simulink model "Power_Model_Official_Pars_2022a"  (R2022a)
settings: Solver=ode23t  StartTime=0.0  StopTime=500  RelTol=1e-3
values from neighbouring files (symbols this model uses):
  anode_tube_D = 0.01    [fuel_cell_battery_par.mat]
  cathode_tube_D = 0.05    [fuel_cell_battery_par.mat]
  comp_rpm_TLU = [0 1800 3600]    [fuel_cell_battery_par.mat]
  coolant_num_layers = 20    [fuel_cell_battery_par.mat]
  coolant_num_passes = 12    [fuel_cell_battery_par.mat]
  coolant_tube_D = 0.05    [fuel_cell_battery_par.mat]
  coolant_w_channels = 1    [fuel_cell_battery_par.mat]
  env_p = 0.101325    [fuel_cell_battery_par.mat]
  env_T = 20    [fuel_cell_battery_par.mat]
  env_yH20 = 0.0115436377169    [fuel_cell_battery_par.mat]
  env_yO2 = 0.21    [fuel_cell_battery_par.mat]
  radiator_air_area_fins = 11.5625    [fuel_cell_battery_par.mat]
  radiator_air_area_primary = 1.223125    [fuel_cell_battery_par.mat]
  radiator_eta_fin = 0.7    [fuel_cell_battery_par.mat]
  radiator_N_tubes = 25    [fuel_cell_battery_par.mat]
  radiator_rho = 2700    [fuel_cell_battery_par.mat]
  radiator_t_wall = 0.0001    [fuel_cell_battery_par.mat]
  radiator_tube_H = 0.0015    [fuel_cell_battery_par.mat]
  radiator_W = 0.025    [fuel_cell_battery_par.mat]
  stack_area = 280    [fuel_cell_battery_par.mat]
  stack_iL = 1.4    [fuel_cell_battery_par.mat]
  stack_mea_rho = 1800    [fuel_cell_battery_par.mat]
  stack_num_cells = 400    [fuel_cell_battery_par.mat]
  stack_num_channels = 8    [fuel_cell_battery_par.mat]
  stack_t_gdl = 250    [fuel_cell_battery_par.mat]
  stack_t_membrane = 125    [fuel_cell_battery_par.mat]
  stack_w_channels = 1    [fuel_cell_battery_par.mat]
undefined symbols (not defined in the file or in its folder): Bat, BattCapInit, BattChargeMax, BattTempBp, CapLUTBp, CapSOCBp, Em, f_fc_auxpower, f_fc_currcmd_bpt, f_fc_h2flow, f_fc_heatflow, f_fc_tmpcmd_bpt, f_fc_voltage, Mot, Np, Ns, RInt, Tc_Batt
libraries: fl_lib x89, nesl_utility x39, FuelCell_lib x32, ee_lib x3, slpidlib x3, batteryecm_lib x1, simulink_extras x1, autolibshared x1, simulink x1
(part 4 of 4)

== system Power_Model_Official_Pars_2022a/Fuel Cell/Fuel Cell/Simscape Fuel Cell_2/Hydrogen Source ==
  Constant1 : Constant  Value=env_p
  Fuel Tank : FuelCell_lib/elements/Constant Volume Chamber (FC)  V0=tank_V l  num_ports=foundation.enum.num_ports.one  area_A=0.01 m^2  area_B=0.01 m^2  area_C=0.01 m^2  area_D=0.01 m^2  cond_spec=FuelCell.enum.ChamberCondSpec.Enabled  tau_c=1 s  is_cond=[0; 0; 0; 0]  out_comp=FuelCell.enum.Composition.Mole  p0=tank_p MPa  T0=env_T degC  comp=FuelCell.enum.Composition.Mole  y0=[0; 0; 1; 0]  x0=[1; 0; 0; 0]
      settings: InternalSimscapePortConfiguration="{\"Bottom\":[{\"id\":\"H\",\"label\":\"H\",\"type\":\"foundation.thermal.thermal\"}],\"Left\":[{\"id\":\"MIn\",\"label\":\"MIn\",\"type\":\"input\"},{\"id\":\"TIn\",\"label\":\"TIn\",\"type\":\"input\"}],\"Right\":[{\"id\":\"pC\",\"label\":\"p\",\"type\":\"output\"},{\"id\":\"TC\",\"label\":\"T\",\"type\":\"output\"},{\"id\":\"yC_i\",\"label\":\"y_i\",\"type\":\"output\"}],\"Top\":[{\"id\":\"A\",\"label\":\"A\",\"type\":\"FuelCell.FuelCell\"}]}"
  Perfect Insulator : fl_lib/Thermal/Thermal Elements/Perfect Insulator  T_specify=off  T_priority=None  T=0 K  T_nominal_specify=off  T_nominal_unit=K  T_nominal_value=1
  Perfect Insulator1 : fl_lib/Thermal/Thermal Elements/Perfect Insulator  T_specify=off  T_priority=None  T=0 K  T_nominal_specify=off  T_nominal_unit=K  T_nominal_value=1
  Pipe (FC) : FuelCell_lib/elements/Pipe (FC)  length=1 m  area=pi*anode_tube_D^2/4 m^2  Dh=anode_tube_D m  extra_length=0.1 * 100 m  roughness=15e-6 m  Re_lam=2000  Re_tur=4000  shape_factor=64  Nu_lam=3.66  tau_c=1e-3 s  isCond=[0; 0; 0; 0]  volMeas=false  compMeas=FuelCell.enum.Composition.Mole  p0=env_p MPa  T0=env_T degC  comp=FuelCell.enum.Composition.Mole  y0=[0; 0; 1; 0]  x0=[1; 0; 0; 0]
      settings: InternalSimscapePortConfiguration="{\"Bottom\":[{\"id\":\"MIn\",\"label\":\"M_in\",\"type\":\"input\"},{\"id\":\"TIn\",\"label\":\"T_in\",\"type\":\"input\"}],\"Left\":[{\"id\":\"A\",\"label\":\"A\",\"type\":\"FuelCell.FuelCell\"},{\"id\":\"H\",\"label\":\"H\",\"type\":\"foundation.thermal.thermal\"}],\"Right\":[{\"id\":\"B\",\"label\":\"B\",\"type\":\"FuelCell.FuelCell\"}],\"Top\":[]}"
  Pressure-Reducing Valve : Subsystem  Tag=PublishSubsystem  mask(Pressure-Reducing Valve){D=anode_tube_D, r_min=1e-4, r_max=0.2, p_range=0.005}
      mask prompts: D "Connecting tube diameter (m)"; r_min "Min diameter ratio"; r_max "Max diameter ratio"; p_range "Pressure regulation range (MPa)"
      mask help: This subsystem models a pressure reducing valve that maintains a set pressure at port B. The valve is normally open. When the pressure is above the set pressure, it is fully closed.
  Simulink-PS Converter : nesl_utility/Simulink-PS Converter  PhysicalDomain=network_engine_domain  SubClassName=ps_input  LeftPortType=input  RightPortType=output  PseudoPeriodic=off  Frequencies=[]  NoiseDistribution=none  NoiseParameters=[]  Unit=MPa  AffineConversion=off  FilteringAndDerivatives=provide  SimscapeFilterOrder=1  InputFilterTimeConstant=0.001  UdotUserProvided=0
  Stack Pressure : Constant  Value=0.06
  Sum : Sum  Inputs=++|
  H2 : PMIOPort  Side=Right
  wires:
  Sum/1 -> Simulink-PS Converter/1
  Constant1/1 -> Sum/2
  Stack Pressure/1 -> Sum/1
  connections:
  Perfect Insulator/LConn1 -- Fuel Tank/RConn4
  Fuel Tank/LConn3 -- Pressure-Reducing Valve/LConn1
  Pressure-Reducing Valve/RConn1 -- Pipe (FC)/LConn1
  Pipe (FC)/RConn1 -- H2/RConn1
  Perfect Insulator1/LConn1 -- Pipe (FC)/LConn2
  Simulink-PS Converter/RConn1 -- Pressure-Reducing Valve/LConn2

== system Power_Model_Official_Pars_2022a/Fuel Cell/Fuel Cell/Simscape Fuel Cell_2/Measurements ==
  Gain : Gain  Gain=1e-3
  Mux : Mux  Inputs=2
  Product : Product
  i : Outport
  v : Outport  Port=2
  P : Outport  Port=3
  T : Outport  Port=4
  wires:
  [v_stack] -> Product/2, v/1
  [i_stack] -> Product/1, i/1
  [T_stack] -> T/1
  [Q_stack] -> Mux/2
  Product/1 -> Gain/1
  Mux/1 -> P/1
  Gain/1 -> Mux/1

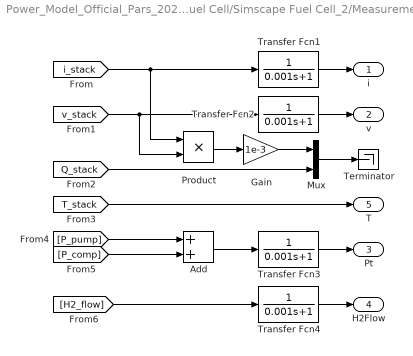
== system Power_Model_Official_Pars_2022a/Fuel Cell/Fuel Cell/Simscape Fuel Cell_2/Measurements1 ==
  Add : Sum
  Gain : Gain  Gain=1e-3
  Mux : Mux  Inputs=2
  Product : Product
  Terminator : Terminator
  Transfer Fcn{1..4} (4 alike) : TransferFcn  Denominator=[0.001 1]
  i : Outport
  v : Outport  Port=2
  Pt : Outport  Port=3
  H2Flow : Outport  Port=4
  T : Outport  Port=5
  wires:
  Gain/1 -> Mux/1
  Mux/1 -> Terminator/1
  Product/1 -> Gain/1
  [Q_stack] -> Mux/2
  [T_stack] -> T/1
  [i_stack] -> Transfer Fcn1/1, Product/1
  [v_stack] -> Transfer Fcn2/1, Product/2
  Transfer Fcn1/1 -> i/1
  Transfer Fcn2/1 -> v/1
  [P_pump] -> Add/1
  [P_comp] -> Add/2
  Add/1 -> Transfer Fcn3/1
  Transfer Fcn3/1 -> Pt/1
  [H2_flow] -> Transfer Fcn4/1
  Transfer Fcn4/1 -> H2Flow/1

== system Power_Model_Official_Pars_2022a/Fuel Cell/Fuel Cell/Simscape Fuel Cell_2/Oxygen Source ==
  i_cmd : Inport
  Air Intake : FuelCell_lib/elements/Reservoir (FC)  constCond=true  p0=env_p MPa  T0=env_T degC  comp=FuelCell.enum.Composition.Mole  y0=[1-env_yO2-env_yH20; env_yO2; 0; env_yH20]  x0=[1; 0; 0; 0]  area=pi*cathode_tube_D^2/4 m^2
      settings: InternalSimscapePortConfiguration="{\"Bottom\":[],\"Left\":[],\"Right\":[],\"Top\":[{\"id\":\"A\",\"label\":\"A\",\"type\":\"FuelCell.FuelCell\"}]}"
  Compressor : FuelCell_lib/sources/Mass Flow Rate Source (FC)  source_type=foundation.enum.constant_controlled.controlled  flow_rate=0 kg/s  power_spec=foundation.enum.power_spec.isentropic  area_A=pi*cathode_tube_D^2/4 m^2  area_B=pi*cathode_tube_D^2/4 m^2  mdot_A_specify=off  mdot_A_priority=None  mdot_A=0.1 kg/s  mdot_A_nominal_specify=off  mdot_A_nominal_unit=kg/s  mdot_A_nominal_value=1  mdot_B_specify=off  mdot_B_priority=None  mdot_B=0.1 kg/s  mdot_B_nominal_specify=off  mdot_B_nominal_unit=kg/s  mdot_B_nominal_value=1  phi_A_specify=off  phi_A_priority=None  phi_A=0 J/s  phi_A_nominal_specify=off  phi_A_nominal_unit=J/s  phi_A_nominal_value=1  phi_B_specify=off  phi_B_priority=None  phi_B=0 J/s  phi_B_nominal_specify=off  phi_B_nominal_unit=J/s  phi_B_nominal_value=1  mdot_A_i_specify=off  mdot_A_i_priority=None  mdot_A_i=[0; 0; 0; 0] kg/s  mdot_A_i_nominal_specify=off  mdot_A_i_nominal_unit=kg/s  mdot_A_i_nominal_value=1  mdot_B_i_specify=off  mdot_B_i_priority=None  mdot_B_i=[0; 0; 0; 0] kg/s  mdot_B_i_nominal_specify=off  mdot_B_i_nominal_unit=kg/s  mdot_B_i_nominal_value=1
      settings: InternalSimscapePortConfiguration="{\"Bottom\":[],\"Left\":[{\"id\":\"M\",\"label\":\"M\",\"type\":\"input\"},{\"id\":\"A\",\"label\":\"A\",\"type\":\"FuelCell.FuelCell\"}],\"Right\":[{\"id\":\"B\",\"label\":\"B\",\"type\":\"FuelCell.FuelCell\"}],\"Top\":[]}"
  Compressor Volume : FuelCell_lib/elements/Constant Volume Chamber (FC)  V0=0.3 l  num_ports=foundation.enum.num_ports.two  area_A=pi*cathode_tube_D^2/4 m^2  area_B=pi*cathode_tube_D^2/4 m^2  area_C=0.01 m^2  area_D=0.01 m^2  cond_spec=FuelCell.enum.ChamberCondSpec.Enabled  tau_c=1e-3 s  is_cond=[0; 0; 0; 0]  out_comp=FuelCell.enum.Composition.Mole  p0=env_p MPa  T0=env_T degC  comp=FuelCell.enum.Composition.Mole  y0=[1-env_yO2-env_yH20; env_yO2; 0; env_yH20]  x0=[1; 0; 0; 0]
      settings: InternalSimscapePortConfiguration="{\"Bottom\":[{\"id\":\"H\",\"label\":\"H\",\"type\":\"foundation.thermal.thermal\"}],\"Left\":[{\"id\":\"MIn\",\"label\":\"MIn\",\"type\":\"input\"},{\"id\":\"TIn\",\"label\":\"TIn\",\"type\":\"input\"}],\"Right\":[{\"id\":\"pC\",\"label\":\"p\",\"type\":\"output\"},{\"id\":\"TC\",\"label\":\"T\",\"type\":\"output\"},{\"id\":\"yC_i\",\"label\":\"y_i\",\"type\":\"output\"}],\"Top\":[{\"id\":\"A\",\"label\":\"A\",\"type\":\"FuelCell.FuelCell\"},{\"id\":\"B\",\"label\":\"B\",\"type\":\"FuelCell.FuelCell\"}]}"
  Compressor Control : Subsystem
  Compressor Map : Subsystem
  Mass Flow Rate Sensor (FC) : FuelCell_lib/sensors/Mass Flow Rate Sensor (FC)
      settings: InternalSimscapePortConfiguration="{\"Bottom\":[],\"Left\":[{\"id\":\"A\",\"label\":\"A\",\"type\":\"FuelCell.FuelCell\"}],\"Right\":[{\"id\":\"M\",\"label\":\"M\",\"type\":\"output\"},{\"id\":\"Phi_out\",\"label\":\"Phi\",\"type\":\"output\"},{\"id\":\"M_i\",\"label\":\"M_i\",\"type\":\"output\"},{\"id\":\"B\",\"label\":\"B\",\"type\":\"FuelCell.FuelCell\"}],\"Top\":[]}"
  Max rpm : fl_lib/Physical Signals/Functions/PS Gain  gain=max(comp_rpm_TLU) rpm
  Oxygen Excess Ratio : Constant  Value=2.5
  PS-Simulink Converter : nesl_utility/PS-Simulink Converter  PhysicalDomain=network_engine_domain  SubClassName=ps_output  LeftPortType=input  RightPortType=output  PseudoPeriodic=off  Frequencies=[]  VectorFormat=1-D array  Unit=kg/s  AffineConversion=off
  Perfect Insulator : fl_lib/Thermal/Thermal Elements/Perfect Insulator  T_specify=off  T_priority=None  T=0 K  T_nominal_specify=off  T_nominal_unit=K  T_nominal_value=1
  Simulink-PS Converter : nesl_utility/Simulink-PS Converter  PhysicalDomain=network_engine_domain  SubClassName=ps_input  LeftPortType=input  RightPortType=output  PseudoPeriodic=off  Frequencies=[]  NoiseDistribution=none  NoiseParameters=[]  Unit=1  AffineConversion=off  FilteringAndDerivatives=provide  SimscapeFilterOrder=1  InputFilterTimeConstant=0.001  UdotUserProvided=0
  O2 : PMIOPort  Side=Left
  wires:
  Compressor Control/1(cmd) -> Simulink-PS Converter/1
  i_cmd/1 -> Compressor Control/2(i)
  PS-Simulink Converter/1 -> Compressor Control/3(M_meas)
  Oxygen Excess Ratio/1 -> Compressor Control/1(OER)
  connections:
  Compressor Map/RConn3 -- Compressor/RConn1 -- Compressor Volume/LConn4
  Compressor Map/RConn1 -- Compressor/LConn2 -- Air Intake/LConn1
  Compressor/LConn1 -- Compressor Map/LConn1
  Simulink-PS Converter/RConn1 -- Max rpm/LConn1
  Max rpm/RConn1 -- Compressor Map/RConn2
  O2/RConn1 -- Mass Flow Rate Sensor (FC)/RConn4
  PS-Simulink Converter/LConn1 -- Mass Flow Rate Sensor (FC)/RConn1
  Compressor Volume/RConn4 -- Perfect Insulator/LConn1
  Compressor Volume/LConn3 -- Mass Flow Rate Sensor (FC)/LConn1

== system Power_Model_Official_Pars_2022a/Fuel Cell/Fuel Cell/Simscape Fuel Cell_2/Recirculation ==
  Constant Volume Chamber (FC) : FuelCell_lib/elements/Constant Volume Chamber (FC)  V0=0.05^3 m^3  num_ports=foundation.enum.num_ports.three  area_A=pi*anode_tube_D^2/4 m^2  area_B=pi*anode_tube_D^2/4 m^2  area_C=pi*anode_tube_D^2/4 m^2  area_D=0.01 m^2  cond_spec=FuelCell.enum.ChamberCondSpec.Enabled  tau_c=1e-3 s  is_cond=[0; 0; 0; 0]  out_comp=FuelCell.enum.Composition.Mole  p0=env_p MPa  T0=env_T degC  comp=FuelCell.enum.Composition.Mole  y0=[0; 0; 1; 0]  x0=[1; 0; 0; 0]
      settings: InternalSimscapePortConfiguration="{\"Bottom\":[{\"id\":\"H\",\"label\":\"H\",\"type\":\"foundation.thermal.thermal\"}],\"Left\":[{\"id\":\"MIn\",\"label\":\"MIn\",\"type\":\"input\"},{\"id\":\"TIn\",\"label\":\"TIn\",\"type\":\"input\"}],\"Right\":[{\"id\":\"pC\",\"label\":\"p\",\"type\":\"output\"},{\"id\":\"TC\",\"label\":\"T\",\"type\":\"output\"},{\"id\":\"yC_i\",\"label\":\"y_i\",\"type\":\"output\"}],\"Top\":[{\"id\":\"A\",\"label\":\"A\",\"type\":\"FuelCell.FuelCell\"},{\"id\":\"B\",\"label\":\"B\",\"type\":\"FuelCell.FuelCell\"},{\"id\":\"C\",\"label\":\"C\",\"type\":\"FuelCell.FuelCell\"}]}"
  Feedforward Control : Subsystem
  Mass Flow Rate Source (FC) : FuelCell_lib/sources/Mass Flow Rate Source (FC)  source_type=foundation.enum.constant_controlled.controlled  flow_rate=0 kg/s  power_spec=foundation.enum.power_spec.none  area_A=0.01 m^2  area_B=0.01 m^2  mdot_A_specify=off  mdot_A_priority=None  mdot_A=0.1 kg/s  mdot_A_nominal_specify=off  mdot_A_nominal_unit=kg/s  mdot_A_nominal_value=1  mdot_B_specify=off  mdot_B_priority=None  mdot_B=0.1 kg/s  mdot_B_nominal_specify=off  mdot_B_nominal_unit=kg/s  mdot_B_nominal_value=1  phi_A_specify=off  phi_A_priority=None  phi_A=0 J/s  phi_A_nominal_specify=off  phi_A_nominal_unit=J/s  phi_A_nominal_value=1  phi_B_specify=off  phi_B_priority=None  phi_B=0 J/s  phi_B_nominal_specify=off  phi_B_nominal_unit=J/s  phi_B_nominal_value=1  mdot_A_i_specify=off  mdot_A_i_priority=None  mdot_A_i=[0; 0; 0; 0] kg/s  mdot_A_i_nominal_specify=off  mdot_A_i_nominal_unit=kg/s  mdot_A_i_nominal_value=1  mdot_B_i_specify=off  mdot_B_i_priority=None  mdot_B_i=[0; 0; 0; 0] kg/s  mdot_B_i_nominal_specify=off  mdot_B_i_nominal_unit=kg/s  mdot_B_i_nominal_value=1
      settings: InternalSimscapePortConfiguration="{\"Bottom\":[],\"Left\":[{\"id\":\"M\",\"label\":\"M\",\"type\":\"input\"},{\"id\":\"A\",\"label\":\"A\",\"type\":\"FuelCell.FuelCell\"}],\"Right\":[{\"id\":\"B\",\"label\":\"B\",\"type\":\"FuelCell.FuelCell\"}],\"Top\":[]}"
  Max Flow : fl_lib/Physical Signals/Functions/PS Gain  gain=0.01 kg/s
  Perfect Insulator : fl_lib/Thermal/Thermal Elements/Perfect Insulator  T_specify=off  T_priority=None  T=0 K  T_nominal_specify=off  T_nominal_unit=K  T_nominal_value=1
  Simulink-PS Converter : nesl_utility/Simulink-PS Converter  PhysicalDomain=network_engine_domain  SubClassName=ps_input  LeftPortType=input  RightPortType=output  PseudoPeriodic=off  Frequencies=[]  NoiseDistribution=none  NoiseParameters=[]  Unit=1  AffineConversion=off  FilteringAndDerivatives=provide  SimscapeFilterOrder=1  InputFilterTimeConstant=0.001  UdotUserProvided=0
  A : PMIOPort  Side=Left
  B : PMIOPort  Port=2  Side=Right
  R : PMIOPort  Port=3  Side=Right
  wires:
  [i_stack] -> Feedforward Control/1(i)
  Feedforward Control/1(cmd) -> Simulink-PS Converter/1
  connections:
  Max Flow/RConn1 -- Mass Flow Rate Source (FC)/LConn1
  Simulink-PS Converter/RConn1 -- Max Flow/LConn1
  R/RConn1 -- Mass Flow Rate Source (FC)/LConn2
  Perfect Insulator/LConn1 -- Constant Volume Chamber (FC)/RConn4
  Constant Volume Chamber (FC)/LConn4 -- Mass Flow Rate Source (FC)/RConn1
  A/RConn1 -- Constant Volume Chamber (FC)/LConn3
  B/RConn1 -- Constant Volume Chamber (FC)/LConn5

== system Power_Model_Official_Pars_2022a/Fuel Cell/Fuel Cell/Simscape Fuel Cell_2/Sensors ==
  Capacitor : fl_lib/Electrical/Electrical Elements/Capacitor  c=1e-6 F  r=1e-6 Ohm  g=0 1/Ohm  i_specify=off  i_priority=None  i=0 A  i_nominal_specify=off  i_nominal_unit=A  i_nominal_value=1  v_specify=off  v_priority=None  v=0 V  v_nominal_specify=off  v_nominal_unit=V  v_nominal_value=1  vc_specify=on  vc_priority=High  vc=f_fc_voltage(1) V  vc_nominal_specify=off  vc_nominal_unit=V  vc_nominal_value=1
  Current Sensor : fl_lib/Electrical/Electrical Sensors/Current Sensor
  Diode : fl_lib/Electrical/Electrical Elements/Diode  Vf=0.6 V  Ron=0.3 Ohm  Goff=1e-8 1/Ohm  i_specify=off  i_priority=None  i=0 A  i_nominal_specify=off  i_nominal_unit=A  i_nominal_value=1  v_specify=off  v_priority=None  v=0 V  v_nominal_specify=off  v_nominal_unit=V  v_nominal_value=1
  PS-Simulink Converter1 : nesl_utility/PS-Simulink Converter  PhysicalDomain=network_engine_domain  SubClassName=ps_output  LeftPortType=input  RightPortType=output  PseudoPeriodic=off  Frequencies=[]  VectorFormat=1-D array  Unit=V  AffineConversion=off
  PS-Simulink Converter2 : nesl_utility/PS-Simulink Converter  PhysicalDomain=network_engine_domain  SubClassName=ps_output  LeftPortType=input  RightPortType=output  PseudoPeriodic=off  Frequencies=[]  VectorFormat=1-D array  Unit=A  AffineConversion=off
  Resistor : fl_lib/Electrical/Electrical Elements/Resistor  R=1e-3 Ohm  i_specify=off  i_priority=None  i=0 A  i_nominal_specify=off  i_nominal_unit=A  i_nominal_value=1  v_specify=off  v_priority=None  v=0 V  v_nominal_specify=off  v_nominal_unit=V  v_nominal_value=1
  Voltage Sensor : fl_lib/Electrical/Electrical Sensors/Voltage Sensor
  + : PMIOPort  Side=Left
  - : PMIOPort  Port=2  Side=Right
  +1 : PMIOPort  Port=3  Side=Left
  -1 : PMIOPort  Port=4  Side=Right
  tag scope: i_stack=global, v_stack=global
  wires:
  PS-Simulink Converter1/1 -> [v_stack]
  PS-Simulink Converter2/1 -> [i_stack]
  connections:
  Capacitor/RConn1 -- -1/RConn1 -- Voltage Sensor/RConn2 -- +1/RConn1
  Capacitor/LConn1 -- Diode/RConn1 -- Current Sensor/LConn1 -- Voltage Sensor/LConn1
  +/RConn1 -- Resistor/LConn1
  Current Sensor/RConn2 -- -/RConn1
  PS-Simulink Converter1/LConn1 -- Voltage Sensor/RConn1
  Resistor/RConn1 -- Diode/LConn1
  PS-Simulink Converter2/LConn1 -- Current Sensor/RConn1

== system Power_Model_Official_Pars_2022a/Fuel Cell/Fuel Cell/Simscape Fuel Cell_2/Subsystem ==
  N2 : Outport
  Purge : Outport  Port=2
  wires:
  [yN2] -> N2/1  "N2 molar fraction"
  [Purge] -> Purge/1  "Purge valve enabled"

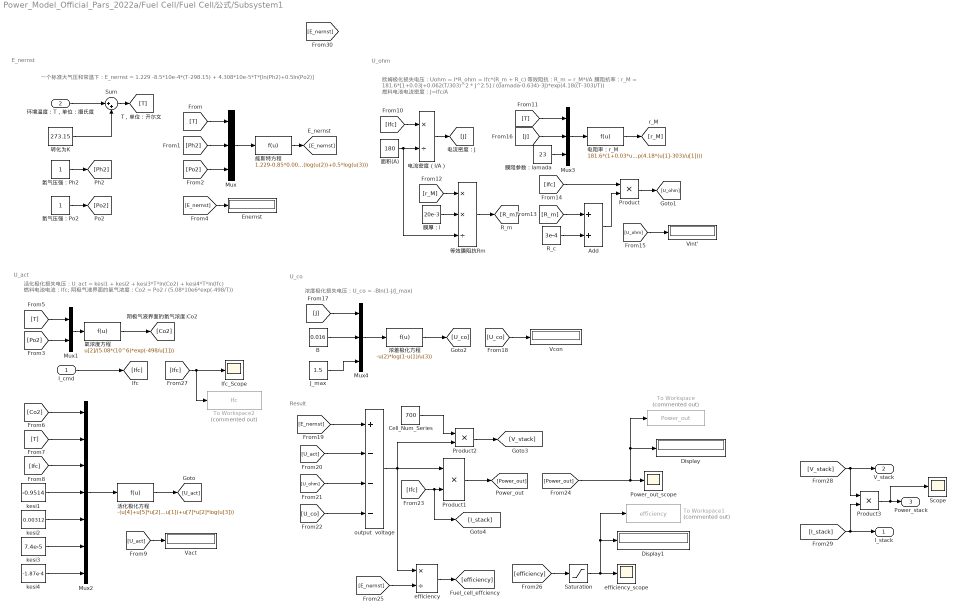
== system Power_Model_Official_Pars_2022a/Fuel Cell/Fuel Cell/公式/Subsystem1 ==
  note: Result
  note: U_co
  note: 浓度极化损失电压：U_co = -Bln(1-J/J_max)
  note: U_ohm
  note: 欧姆极化损失电压：Uohm = I*R_ohm = Ifc*(R_m + R_c)
      | 等效阻抗：R_m = r_M*l/A
      | 膜阻抗率：r_M = 181.6*[1+0.03J+0.062(T/303)^2 * J^2.5] / ((lamada-0.634)-3J)*exp(4.18((T-303)/T))
      | 燃料电池电流密度：J=Ifc/A
  note: U_act
  note: 活化极化损失电压：U_act = kesi1 + kesi2 + kesi3*T*ln(Co2) + kesi4*T*ln(Ifc)
      | 燃料电池电流：Ifc;
      | 阴极气液界面的氧气浓度：Co2 = Po2 / (5.08*10e6*exp(-498/T))
  note: E_nernst
  note: 一个标准大气压和常温下：E_nernst = 1.229 -8.5*10e-4*(T-298.15) + 4.308*10e-5*T*[ln(Ph2)+0.5ln(Po2)]
  I_cmd : Inport
  环境温度：T，单位：摄氏度 : Inport  Port=2
  Add : Sum
  B : Constant  Value=0.016
  Cell_Num_Series : Constant  Value=700
  Display : Display
  Display1 : Display
  Enernst : Display
      settings: Decimation=5
  Ifc_Scope : Scope
  J_max : Constant  Value=1.5
  Mux : Mux  Inputs=3
  Mux1 : Mux  Inputs=2
  Mux2 : Mux  Inputs=7
  Mux3 : Mux  Inputs=3
  Mux4 : Mux  Inputs=3
  Power_out_scope : Scope
  Product{,1..3} (4 alike) : Product
  R_c : Constant  Value=3e-4
  Saturation : Saturate  UpperLimit=0.9  LowerLimit=0
  Scope : Scope
  Sum : Sum  Inputs=|++
  To Workspace : ToWorkspace  Commented=on  VariableName=Power_out  SampleTime=-1
      settings: Save2DSignal=2-D array (concatenate along first dimension)
  To Workspace1 : ToWorkspace  Commented=on  VariableName=efficiency  SampleTime=-1
      settings: Save2DSignal=2-D array (concatenate along first dimension)
  To Workspace2 : ToWorkspace  Commented=on  VariableName=Ifc  SampleTime=-1
      settings: Save2DSignal=2-D array (concatenate along first dimension)
  Vact : Display
      settings: Decimation=5
  Vcon : Display
      settings: Decimation=5
  Vint' : Display
      settings: Decimation=5
  efficiency : Product  Inputs=*/  OutDataTypeStr=double
  efficiency_scope : Scope
  kesi1 : Constant  Value=-0.9514
  kesi2 : Constant  Value=0.00312
  kesi3 : Constant  Value=7.4e-5
  kesi4 : Constant  Value=-1.87e-4
  output  voltage : Sum  Inputs=+---  OutDataTypeStr=double
  氢气压强：Ph2 : Constant
  氧气压强：Po2 : Constant
  氧浓度方程 : Fcn  Expr=u[2]/(5.08*(10^6)*exp(-498/u[1]))
  活化极化方程 : Fcn  Expr=-(u[4]+u[5]*u[2]+u[6]*u[2]*log(u[1])+u[7]*u[2]*log(u[3]))
  浓差极化方程 : Fcn  Expr=-u(2)*log(1-u(1)/u(3))
  电流密度（I/A） : Product  Inputs=*/  OutDataTypeStr=double
  电阻率：r_M : Fcn  Expr=181.6*(1+0.03*u[2]+0.062*((u[1]/303)^2)*(u[2]^2.5))/((u[3]-0.634-3*u[2])*(exp(4.18*(u[1]-303)/u[1])))
  等效膜阻抗Rm : Product  Inputs=**/  OutDataTypeStr=double
  能斯特方程 : Fcn  Expr=1.229-0.85*0.001*(u(1)-298.15)+4.3085*0.00001*u(1)*(log(u(2))+0.5*log(u(3)))
  膜厚：l : Constant  Value=20e-3
  膜阻参数：lamada : Constant  Value=23
  转化为K : Constant  Value=273.15
  面积(A) : Constant  Value=180
  I_stack : Outport
  V_stack : Outport  Port=2
  Power_stack : Outport  Port=3
  wires:
  [E_nernst] -> efficiency/2
  环境温度：T，单位：摄氏度/1 -> Sum/1
  [T] -> Mux/1
  Sum/1 -> [T]
  [Ifc] -> 电流密度（I/A）/1
  [Co2] -> Mux2/1
  Mux2/1 -> 活化极化方程/1
  [T] -> Mux2/2
  转化为K/1 -> Sum/2
  能斯特方程/1 -> [E_nernst]
  [Ifc] -> To Workspace2/1, Ifc_Scope/1
  Saturation/1 -> efficiency_scope/1, To Workspace1/1, Display1/1
  面积(A)/1 -> 电流密度（I/A）/2, 等效膜阻抗Rm/3
  [T] -> Mux1/1
  活化极化方程/1 -> [U_act]
  电流密度（I/A）/1 -> [J]
  output  voltage/1 -> Product2/2, efficiency/1, Product1/1
  [U_act] -> output  voltage/2
  氧气压强：Po2/1 -> [Po2]
  [r_M] -> 等效膜阻抗Rm/1
  氢气压强：Ph2/1 -> [Ph2]
  [Ifc] -> Product/1
  等效膜阻抗Rm/1 -> [R_m]
  efficiency/1 -> [efficiency]
  R_c/1 -> Add/2
  Mux4/1 -> 浓差极化方程/1
  [E_nernst] -> Enernst/1
  [Ph2] -> Mux/2
  kesi2/1 -> Mux2/5
  J_max/1 -> Mux4/3
  膜厚：l/1 -> 等效膜阻抗Rm/2
  [efficiency] -> Saturation/1
  [R_m] -> Add/1
  [U_co] -> Vcon/1
  [Power_out] -> Power_out_scope/1, To Workspace/1, Display/1
  Product1/1 -> [Power_out]
  [J] -> Mux4/1
  [U_ohm] -> output  voltage/3
  Cell_Num_Series/1 -> Product2/1
  浓差极化方程/1 -> [U_co]
  [V_stack] -> V_stack/1, Product3/1
  kesi1/1 -> Mux2/4
  kesi4/1 -> Mux2/7
  [U_act] -> Vact/1
  Mux1/1 -> 氧浓度方程/1
  Mux/1 -> 能斯特方程/1
  [Po2] -> Mux1/2
  膜阻参数：lamada/1 -> Mux3/3
  [Po2] -> Mux/3
  kesi3/1 -> Mux2/6
  [I_stack] -> I_stack/1, Product3/2
  [U_ohm] -> Vint'/1
  氧浓度方程/1 -> [Co2]
  B/1 -> Mux4/2
  Mux3/1 -> 电阻率：r_M/1
  [T] -> Mux3/1
  电阻率：r_M/1 -> [r_M]
  Add/1 -> Product/2
  [E_nernst] -> output  voltage/1
  [Ifc] -> Mux2/3
  [Ifc] -> [I_stack], Product1/2
  [J] -> Mux3/2
  [U_co] -> output  voltage/4
  Product/1 -> [U_ohm]
  Product3/1 -> Scope/1, Power_stack/1
  I_cmd/1 -> [Ifc]
  Product2/1 -> [V_stack]

== system Power_Model_Official_Pars_2022a/Fuel Cell/Fuel Cell/Simscape Fuel Cell_2/Anode Humidifier/Proportional Control ==
  RH_set : Inport
  RH_meas : Inport  Port=2
  Gain : Gain  Gain=0.1
  Saturation : Saturate  UpperLimit=inf  LowerLimit=0  ZeroCross=off
  Selector : Selector  InputPortWidth=4  IndexOptions=Index vector (dialog)  Indices=[4]  OutputSizes=1
  Sum : Sum  Inputs=|+-
  Transfer Fcn : TransferFcn  Denominator=[1 1]
  Mw : Outport
  wires:
  Saturation/1 -> Transfer Fcn/1
  RH_meas/1 -> Selector/1
  RH_set/1 -> Sum/1
  Sum/1 -> Gain/1
  Gain/1 -> Saturation/1
  Transfer Fcn/1 -> Mw/1
  Selector/1 -> Sum/2

== system Power_Model_Official_Pars_2022a/Fuel Cell/Fuel Cell/Simscape Fuel Cell_2/Cathode Humidifier/Proportional Control ==
  RH_set : Inport
  RH_meas : Inport  Port=2
  Gain : Gain  Gain=0.1
  Saturation : Saturate  UpperLimit=inf  LowerLimit=0  ZeroCross=off
  Selector : Selector  InputPortWidth=4  IndexOptions=Index vector (dialog)  Indices=[4]  OutputSizes=1
  Sum : Sum  Inputs=|+-
  Transfer Fcn : TransferFcn  Denominator=[1 1]
  Mw : Outport
  wires:
  Saturation/1 -> Transfer Fcn/1
  Gain/1 -> Saturation/1
  Transfer Fcn/1 -> Mw/1
  RH_meas/1 -> Selector/1
  Sum/1 -> Gain/1
  RH_set/1 -> Sum/1
  Selector/1 -> Sum/2

== system Power_Model_Official_Pars_2022a/Fuel Cell/Fuel Cell/Simscape Fuel Cell_2/Cathode Exhaust/Pressure Relief Valve ==
  Absolute Reference (FC) : FuelCell_lib/elements/Absolute Reference (FC)
      settings: InternalSimscapePortConfiguration="{\"Bottom\":[],\"Left\":[{\"id\":\"A\",\"label\":\"\",\"type\":\"FuelCell.FuelCell\"}],\"Right\":[],\"Top\":[]}"
  PS Add : fl_lib/Physical Signals/Functions/PS Add
  PS Constant : fl_lib/Physical Signals/Sources/PS Constant  constant=r_min^2
  PS Gain : fl_lib/Physical Signals/Functions/PS Gain  gain=(r_max^2 - r_min^2)/p_range 1/MPa
  PS Gain1 : fl_lib/Physical Signals/Functions/PS Gain  gain=pi*D^2/4 m^2
  PS Subtract : fl_lib/Physical Signals/Functions/PS Subtract
  Pressure and Temperature Sensor (FC) : FuelCell_lib/sensors/Pressure and Temperature Sensor (FC)
      settings: InternalSimscapePortConfiguration="{\"Bottom\":[],\"Left\":[{\"id\":\"A\",\"label\":\"A\",\"type\":\"FuelCell.FuelCell\"}],\"Right\":[{\"id\":\"P\",\"label\":\"P\",\"type\":\"output\"},{\"id\":\"T\",\"label\":\"T\",\"type\":\"output\"},{\"id\":\"B\",\"label\":\"B\",\"type\":\"FuelCell.FuelCell\"}],\"Top\":[]}"
  Valve : FuelCell_lib/elements/Local Restriction (FC)  const_area=false  restriction_area=0.001 m^2  min_area=pi*(r_min*D)^2/4 m^2  max_area=pi*(r_max*D)^2/4 m^2  area=pi*D^2/4 m^2  Cd=0.64  B_lam=0.999
      settings: InternalSimscapePortConfiguration="{\"Bottom\":[],\"Left\":[{\"id\":\"AR\",\"label\":\"AR\",\"type\":\"input\"},{\"id\":\"A\",\"label\":\"A\",\"type\":\"FuelCell.FuelCell\"}],\"Right\":[{\"id\":\"B\",\"label\":\"B\",\"type\":\"FuelCell.FuelCell\"}],\"Top\":[]}"
  A : PMIOPort  Side=Left
  B : PMIOPort  Port=2  Side=Right
  p_set : PMIOPort  Port=3  Side=Left
  connections:
  PS Add/RConn1 -- PS Gain1/LConn1
  PS Gain/LConn1 -- PS Subtract/RConn1
  PS Gain1/RConn1 -- Valve/LConn1
  Valve/RConn1 -- B/RConn1
  A/RConn1 -- Pressure and Temperature Sensor (FC)/LConn1 -- Valve/LConn2
  PS Gain/RConn1 -- PS Add/LConn1
  PS Add/LConn2 -- PS Constant/RConn1
  p_set/RConn1 -- PS Subtract/LConn2
  Pressure and Temperature Sensor (FC)/RConn1 -- PS Subtract/LConn1
  Absolute Reference (FC)/LConn1 -- Pressure and Temperature Sensor (FC)/RConn3

== system Power_Model_Official_Pars_2022a/Fuel Cell/Fuel Cell/Simscape Fuel Cell_2/Cooling System/Coolant Tank ==
  Coolant Volume : fl_lib/Thermal Liquid/Elements/Translational Mechanical Converter (TL)  mech_orientation=foundation.enum.MechOrientationTranslational.Positive  displacement_spec=foundation.enum.DisplacementSpec.Calculate  x0=x_init m  interface_area=A m^2  dead_volume=A * 0.001 m^3  environment_spec=foundation.enum.pressure_spec.atmospheric  environment_pressure=0.101325 MPa  dynamic_compressibility=simscape.enum.onoff.off  p0=env_p MPa  T0=env_T degC
      settings: InternalSimscapePortConfiguration="{\"Bottom\":[],\"Left\":[{\"id\":\"A\",\"label\":\"A\",\"type\":\"foundation.thermal_liquid.thermal_liquid\"},{\"id\":\"C\",\"label\":\"C\",\"type\":\"foundation.mechanical.translational.translational\"},{\"id\":\"H\",\"label\":\"H\",\"type\":\"foundation.thermal.thermal\"}],\"Right\":[{\"id\":\"R\",\"label\":\"R\",\"type\":\"foundation.mechanical.translational.translational\"}],\"Top\":[]}"
  Mechanical Translational Reference : fl_lib/Mechanical/Translational Elements/Mechanical Translational Reference
  Perfect Insulator : fl_lib/Thermal/Thermal Elements/Perfect Insulator  T_specify=off  T_priority=None  T=0 K  T_nominal_specify=off  T_nominal_unit=K  T_nominal_value=1
  Translational Free End : fl_lib/Mechanical/Translational Elements/Translational Free End  v_specify=off  v_priority=None  v=0 m/s  v_nominal_specify=off  v_nominal_unit=m/s  v_nominal_value=1
      settings: InternalSimscapePortConfiguration="{\"Bottom\":[],\"Left\":[{\"id\":\"V\",\"label\":\"\",\"type\":\"foundation.mechanical.translational.translational\"}],\"Right\":[],\"Top\":[]}"
  T : PMIOPort  Side=Right
  connections:
  Coolant Volume/LConn1 -- T/RConn1
  Mechanical Translational Reference/LConn1 -- Coolant Volume/LConn2
  Translational Free End/LConn1 -- Coolant Volume/RConn1
  Perfect Insulator/LConn1 -- Coolant Volume/LConn3

== system Power_Model_Official_Pars_2022a/Fuel Cell/Fuel Cell/Simscape Fuel Cell_2/Cooling System/Pump Control ==
  T_set : Inport
  T_meas : Inport  Port=2
  Control Signals : Scope  NumInputPorts=2
  Mux : Mux  Inputs=2
  Mux1 : Mux  Inputs=2
  PID Controller : slpidlib/PID Controller  Controller=PI  Form=Ideal  TimeDomain=Continuous-time  UseExternalTs=off  SampleTime=-1  IntegratorMethod=Forward Euler  FilterMethod=Forward Euler  ControllerParametersSource=internal  P=0.1  I=0.01  UseKiTs=off  D=0  N=100  UseFilter=on  TunerSelectOption=Transfer Function Based (PID Tuner App)  InitialConditionSource=internal  InitialConditionForIntegrator=0  InitialConditionForFilter=0  DifferentiatorICPrevScaledInput=0  ExternalReset=none  TrackingMode=off  Kt=1  LimitOutput=on  SatLimitsSource=internal  UpperSaturationLimit=1  LowerSaturationLimit=0  LinearizeAsGain=on  AntiWindupMode=back-calculation  Kb=0.1  POutMin=[]  POutMax=[]  IOutMin=[]  IOutMax=[]  DOutMin=[]  DOutMax=[]  NOutMin=[]  NOutMax=[]  SumOutMin=[]  SumOutMax=[]  SaturationOutMin=[]  SaturationOutMax=[]  PParamMin=[]  PParamMax=[]  IParamMin=[]  IParamMax=[]  DParamMin=[]  DParamMax=[]  NParamMin=[]  NParamMax=[]  KbParamMin=[]  KbParamMax=[]  KtParamMin=[]  KtParamMax=[]  KbOutMin=[]  KbOutMax=[]  KtOutMin=[]  KtOutMax=[]  IntegratorOutMin=[]  IntegratorOutMax=[]  FilterOutMin=[]  FilterOutMax=[]  SumI1OutMin=[]  SumI1OutMax=[]  SumI2OutMin=[]  SumI2OutMax=[]  SumI3OutMin=[]  SumI3OutMax=[]  SumI4OutMin=[]  SumI4OutMax=[]  SumDOutMin=[]  SumDOutMax=[]  DifferentiatorOutMin=[]  DifferentiatorOutMax=[]  FilterDiffOutCoefMin=[]  FilterDiffOutCoefMax=[]  ReciprocalOutMin=[]  ReciprocalOutMax=[]  SumDenOutMin=[]  SumDenOutMax=[]  SumNumOutMin=[]  SumNumOutMax=[]  DivideOutMin=[]  DivideOutMax=[]  UdiffTsProdOutMin=[]  UdiffTsProdOutMax=[]  NTsProdOutMin=[]  NTsProdOutMax=[]  UintegralTsProdOutMin=[]  UintegralTsProdOutMax=[]  UngainTsProdOutMin=[]  UngainTsProdOutMax=[]  IntegratorContinuousStateAttributes=''  IntegratorStateMustResolveToSignalObject=off  IntegratorRTWStateStorageClass=Auto  FilterContinuousStateAttributes=''  FilterStateMustResolveToSignalObject=off  FilterRTWStateStorageClass=Auto  ParallelPVariant=Passthrough  IdealPVariant=InternalParameters  IVariant=InternalParameters  DVariant=Disabled  IntegratorVariant=Continuous  SatVariant=Enabled  AWVariant=BackCalculation  PCopyVariant=Disabled  TRVariant=Disabled  FdbkBlocksVariant=Forward  IdealPFdbkVariant=Disabled  SatFdbkVariant=Disabled  DerivativeFilterVariant=Disabled  NVariant=Disabled  NCopyVariant=Disabled_SignalSpec  FilterICVariant=Disabled  IntegratorICVariant=InternalICs  ExternalResetVariant=Disabled  TRSumVariant=Passthrough  SumFdbkVariant=Disabled  SumVariant=Sum_PI  TsampFilterVariant=InternalTs  TsampNgainVariant=Passthrough  TsampIntegralVariant=Disabled_SignalSpec  ExternalSaturationOutDataTypeStr=Inherit: Same as second input
  Sum : Sum  Inputs=|-+
  Transfer Fcn : TransferFcn  Denominator=[2 1]
  cmd : Outport
  wires:
  Transfer Fcn/1 -> Mux1/2, cmd/1
  T_set/1 -> Mux/1, Sum/1
  T_meas/1 -> Mux/2, Sum/2
  Sum/1 -> PID Controller/1
  PID Controller/1 -> Mux1/1, Transfer Fcn/1
  Mux/1 -> Control Signals/1
  Mux1/1 -> Control Signals/2

== system Power_Model_Official_Pars_2022a/Fuel Cell/Fuel Cell/Simscape Fuel Cell_2/Hydrogen Source/Pressure-Reducing Valve ==
  Absolute Reference (FC) : FuelCell_lib/elements/Absolute Reference (FC)
      settings: InternalSimscapePortConfiguration="{\"Bottom\":[],\"Left\":[{\"id\":\"A\",\"label\":\"\",\"type\":\"FuelCell.FuelCell\"}],\"Right\":[],\"Top\":[]}"
  PS Add : fl_lib/Physical Signals/Functions/PS Add
  PS Constant : fl_lib/Physical Signals/Sources/PS Constant  constant=r_max^2
  PS Constant1 : fl_lib/Physical Signals/Sources/PS Constant  constant=p_range MPa
  PS Gain : fl_lib/Physical Signals/Functions/PS Gain  gain=(r_min^2 - r_max^2)/p_range 1/MPa
  PS Gain1 : fl_lib/Physical Signals/Functions/PS Gain  gain=pi*D^2/4 m^2
  PS Subtract : fl_lib/Physical Signals/Functions/PS Subtract
  PS Subtract1 : fl_lib/Physical Signals/Functions/PS Subtract
  Pressure and Temperature Sensor (FC) : FuelCell_lib/sensors/Pressure and Temperature Sensor (FC)
      settings: InternalSimscapePortConfiguration="{\"Bottom\":[],\"Left\":[{\"id\":\"A\",\"label\":\"A\",\"type\":\"FuelCell.FuelCell\"}],\"Right\":[{\"id\":\"P\",\"label\":\"P\",\"type\":\"output\"},{\"id\":\"T\",\"label\":\"T\",\"type\":\"output\"},{\"id\":\"B\",\"label\":\"B\",\"type\":\"FuelCell.FuelCell\"}],\"Top\":[]}"
  Valve : FuelCell_lib/elements/Local Restriction (FC)  const_area=false  restriction_area=0.001 m^2  min_area=pi*(r_min*D)^2/4 m^2  max_area=pi*(r_max*D)^2/4 m^2  area=pi*D^2/4 m^2  Cd=0.64  B_lam=0.999
      settings: InternalSimscapePortConfiguration="{\"Bottom\":[],\"Left\":[{\"id\":\"AR\",\"label\":\"AR\",\"type\":\"input\"},{\"id\":\"A\",\"label\":\"A\",\"type\":\"FuelCell.FuelCell\"}],\"Right\":[{\"id\":\"B\",\"label\":\"B\",\"type\":\"FuelCell.FuelCell\"}],\"Top\":[]}"
  A : PMIOPort  Side=Left
  B : PMIOPort  Port=2  Side=Right
  p_set : PMIOPort  Port=3  Side=Left
  connections:
  PS Constant1/RConn1 -- PS Subtract1/LConn2
  PS Subtract1/LConn1 -- p_set/RConn1
  PS Subtract1/RConn1 -- PS Subtract/LConn2
  PS Constant/RConn1 -- PS Add/LConn1
  PS Add/LConn2 -- PS Gain/RConn1
  PS Add/RConn1 -- PS Gain1/LConn1
  PS Gain/LConn1 -- PS Subtract/RConn1
  PS Subtract/LConn1 -- Pressure and Temperature Sensor (FC)/RConn1
  PS Gain1/RConn1 -- Valve/LConn1
  Valve/LConn2 -- A/RConn1
  Valve/RConn1 -- B/RConn1 -- Pressure and Temperature Sensor (FC)/LConn1
  Absolute Reference (FC)/LConn1 -- Pressure and Temperature Sensor (FC)/RConn3

== system Power_Model_Official_Pars_2022a/Fuel Cell/Fuel Cell/Simscape Fuel Cell_2/Oxygen Source/Compressor Control ==
  OER : Inport
  i : Inport  Port=2
  M_meas : Inport  Port=3
  Constant : Constant  Value=0.1 * stack_iL * stack_area
  Control Signals : Scope  NumInputPorts=2
  M_set : Gain  Gain=stack_num_cells * 32e-3 / (4*96485) / 0.234
  Max : MinMax  Function=max  Inputs=2  ZeroCross=off
  Mux : Mux  Inputs=2
  Mux1 : Mux  Inputs=2
  PID Controller : slpidlib/PID Controller  Controller=PI  Form=Ideal  TimeDomain=Continuous-time  UseExternalTs=off  SampleTime=-1  IntegratorMethod=Forward Euler  FilterMethod=Forward Euler  ControllerParametersSource=internal  P=5  I=0.5  UseKiTs=off  D=0  N=100  UseFilter=on  TunerSelectOption=Transfer Function Based (PID Tuner App)  InitialConditionSource=internal  InitialConditionForIntegrator=0  InitialConditionForFilter=0  DifferentiatorICPrevScaledInput=0  ExternalReset=none  TrackingMode=off  Kt=1  LimitOutput=on  SatLimitsSource=internal  UpperSaturationLimit=1  LowerSaturationLimit=0  LinearizeAsGain=on  AntiWindupMode=back-calculation  Kb=1  POutMin=[]  POutMax=[]  IOutMin=[]  IOutMax=[]  DOutMin=[]  DOutMax=[]  NOutMin=[]  NOutMax=[]  SumOutMin=[]  SumOutMax=[]  SaturationOutMin=[]  SaturationOutMax=[]  PParamMin=[]  PParamMax=[]  IParamMin=[]  IParamMax=[]  DParamMin=[]  DParamMax=[]  NParamMin=[]  NParamMax=[]  KbParamMin=[]  KbParamMax=[]  KtParamMin=[]  KtParamMax=[]  KbOutMin=[]  KbOutMax=[]  KtOutMin=[]  KtOutMax=[]  IntegratorOutMin=[]  IntegratorOutMax=[]  FilterOutMin=[]  FilterOutMax=[]  SumI1OutMin=[]  SumI1OutMax=[]  SumI2OutMin=[]  SumI2OutMax=[]  SumI3OutMin=[]  SumI3OutMax=[]  SumI4OutMin=[]  SumI4OutMax=[]  SumDOutMin=[]  SumDOutMax=[]  DifferentiatorOutMin=[]  DifferentiatorOutMax=[]  FilterDiffOutCoefMin=[]  FilterDiffOutCoefMax=[]  ReciprocalOutMin=[]  ReciprocalOutMax=[]  SumDenOutMin=[]  SumDenOutMax=[]  SumNumOutMin=[]  SumNumOutMax=[]  DivideOutMin=[]  DivideOutMax=[]  UdiffTsProdOutMin=[]  UdiffTsProdOutMax=[]  NTsProdOutMin=[]  NTsProdOutMax=[]  UintegralTsProdOutMin=[]  UintegralTsProdOutMax=[]  UngainTsProdOutMin=[]  UngainTsProdOutMax=[]  IntegratorContinuousStateAttributes=''  IntegratorStateMustResolveToSignalObject=off  IntegratorRTWStateStorageClass=Auto  FilterContinuousStateAttributes=''  FilterStateMustResolveToSignalObject=off  FilterRTWStateStorageClass=Auto  ParallelPVariant=Passthrough  IdealPVariant=InternalParameters  IVariant=InternalParameters  DVariant=Disabled  IntegratorVariant=Continuous  SatVariant=Enabled  AWVariant=BackCalculation  PCopyVariant=Disabled  TRVariant=Disabled  FdbkBlocksVariant=Forward  IdealPFdbkVariant=Disabled  SatFdbkVariant=Disabled  DerivativeFilterVariant=Disabled  NVariant=Disabled  NCopyVariant=Disabled_SignalSpec  FilterICVariant=Disabled  IntegratorICVariant=InternalICs  ExternalResetVariant=Disabled  TRSumVariant=Passthrough  SumFdbkVariant=Disabled  SumVariant=Sum_PI  TsampFilterVariant=InternalTs  TsampNgainVariant=Passthrough  TsampIntegralVariant=Disabled_SignalSpec  ExternalSaturationOutDataTypeStr=Inherit: Same as second input
  Product : Product
  Sum : Sum  Inputs=|+-
  Transfer Fcn : TransferFcn  Denominator=[2 1]
  cmd : Outport
  wires:
  OER/1 -> Product/1
  Constant/1 -> Max/2
  i/1 -> Max/1
  Max/1 -> Product/2
  PID Controller/1 -> Mux1/1, Transfer Fcn/1
  Sum/1 -> PID Controller/1
  M_set/1 -> Sum/1, Mux/1
  Product/1 -> M_set/1
  M_meas/1 -> Mux/2, Sum/2
  Transfer Fcn/1 -> Mux1/2, cmd/1
  Mux/1 -> Control Signals/1
  Mux1/1 -> Control Signals/2

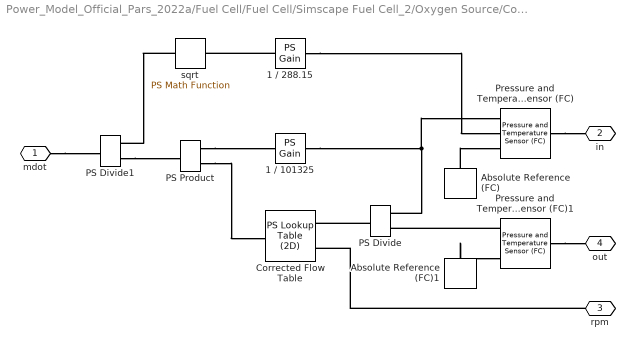
== system Power_Model_Official_Pars_2022a/Fuel Cell/Fuel Cell/Simscape Fuel Cell_2/Oxygen Source/Compressor Map ==
  1 / 101325 : fl_lib/Physical Signals/Functions/PS Gain  gain=1 / 101325 1/Pa
  1 / 288.15 : fl_lib/Physical Signals/Functions/PS Gain  gain=1 / 288.15 1/K
  Absolute Reference (FC) : FuelCell_lib/elements/Absolute Reference (FC)
      settings: InternalSimscapePortConfiguration="{\"Bottom\":[],\"Left\":[{\"id\":\"A\",\"label\":\"\",\"type\":\"FuelCell.FuelCell\"}],\"Right\":[],\"Top\":[]}"
  Absolute Reference (FC)1 : FuelCell_lib/elements/Absolute Reference (FC)
      settings: InternalSimscapePortConfiguration="{\"Bottom\":[],\"Left\":[{\"id\":\"A\",\"label\":\"\",\"type\":\"FuelCell.FuelCell\"}],\"Right\":[],\"Top\":[]}"
  Corrected Flow Table : fl_lib/Physical Signals/Lookup Tables/PS Lookup Table (2D)  x1=comp_p_ratio_TLU Pa/Pa  x2=comp_rpm_TLU rpm  f=comp_mdot_corr_TLU kg/s  interp_method=simscape.enum.interpolation.linear  extrap_method=simscape.enum.extrapolation.nearest
  PS Divide : fl_lib/Physical Signals/Functions/PS Divide
  PS Divide1 : fl_lib/Physical Signals/Functions/PS Divide
  PS Product : fl_lib/Physical Signals/Functions/PS Product
  Pressure and Temperature Sensor (FC) : FuelCell_lib/sensors/Pressure and Temperature Sensor (FC)
      settings: InternalSimscapePortConfiguration="{\"Bottom\":[],\"Left\":[{\"id\":\"A\",\"label\":\"A\",\"type\":\"FuelCell.FuelCell\"}],\"Right\":[{\"id\":\"P\",\"label\":\"P\",\"type\":\"output\"},{\"id\":\"T\",\"label\":\"T\",\"type\":\"output\"},{\"id\":\"B\",\"label\":\"B\",\"type\":\"FuelCell.FuelCell\"}],\"Top\":[]}"
  Pressure and Temperature Sensor (FC)1 : FuelCell_lib/sensors/Pressure and Temperature Sensor (FC)
      settings: InternalSimscapePortConfiguration="{\"Bottom\":[],\"Left\":[{\"id\":\"A\",\"label\":\"A\",\"type\":\"FuelCell.FuelCell\"}],\"Right\":[{\"id\":\"P\",\"label\":\"P\",\"type\":\"output\"},{\"id\":\"T\",\"label\":\"T\",\"type\":\"output\"},{\"id\":\"B\",\"label\":\"B\",\"type\":\"FuelCell.FuelCell\"}],\"Top\":[]}"
  sqrt : fl_lib/Physical Signals/Functions/PS Math Function  fcn_choice=foundation.enum.math_function.sqrt  v=1
  mdot : PMIOPort  Side=Left
  in : PMIOPort  Port=2  Side=Right
  rpm : PMIOPort  Port=3  Side=Right
  out : PMIOPort  Port=4  Side=Right
  connections:
  1 / 101325/LConn1 -- Pressure and Temperature Sensor (FC)/RConn1 -- PS Divide/LConn2
  rpm/RConn1 -- Corrected Flow Table/LConn2
  PS Divide/RConn1 -- Corrected Flow Table/LConn1
  1 / 288.15/LConn1 -- Pressure and Temperature Sensor (FC)/RConn2
  PS Product/LConn1 -- 1 / 101325/RConn1
  PS Product/LConn2 -- Corrected Flow Table/RConn1
  PS Divide1/LConn1 -- PS Product/RConn1
  1 / 288.15/RConn1 -- sqrt/LConn1
  sqrt/RConn1 -- PS Divide1/LConn2
  mdot/RConn1 -- PS Divide1/RConn1
  Pressure and Temperature Sensor (FC)1/RConn1 -- PS Divide/LConn1
  Absolute Reference (FC)/LConn1 -- Pressure and Temperature Sensor (FC)/RConn3
  Pressure and Temperature Sensor (FC)/LConn1 -- in/RConn1
  Absolute Reference (FC)1/LConn1 -- Pressure and Temperature Sensor (FC)1/RConn3
  Pressure and Temperature Sensor (FC)1/LConn1 -- out/RConn1

== system Power_Model_Official_Pars_2022a/Fuel Cell/Fuel Cell/Simscape Fuel Cell_2/Recirculation/Feedforward Control ==
  i : Inport
  Constant : Constant  Value=0.2
  Gain : Gain  Gain=0.8 / (stack_iL * stack_area)
  Saturation : Saturate  UpperLimit=1  LowerLimit=0
  Sum : Sum  Inputs=|++
  Transfer Fcn : TransferFcn  Denominator=[2 1]
  cmd : Outport
  wires:
  i/1 -> Gain/1
  Transfer Fcn/1 -> cmd/1
  Gain/1 -> Sum/1
  Constant/1 -> Sum/2
  Sum/1 -> Saturation/1
  Saturation/1 -> Transfer Fcn/1
